simulink model "LAB2_1"  (R2025b)
settings: Solver=FixedStepAuto  StartTime=0.0  StopTime=5  FixedStep=0.0001  RelTol=1e-3
undefined symbols (not defined in the file): Beq, daq, DiscIntNeverNeededParam, drv, gbox, Jeq, Kd, Kp, mot, rads2rpm, Req, sens, T, tau_sf_est, Tl
settings Model: Creator=Gioele  LastModifiedBy=Gioele
settings DebuggingCC: MultiTaskCondExecSysMsg=warning  MultiTaskRateTransMsg=warning

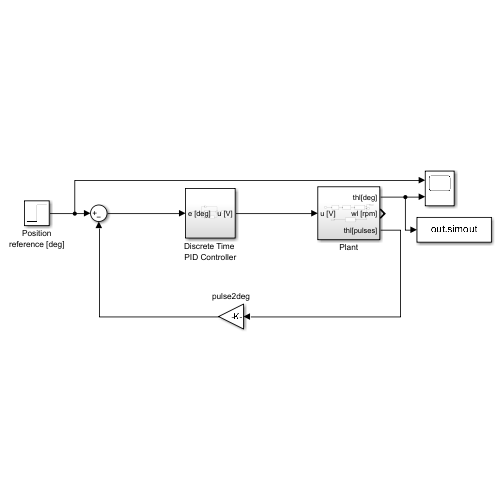
[thumbnail: Simulink's stored preview of the top-level diagram]
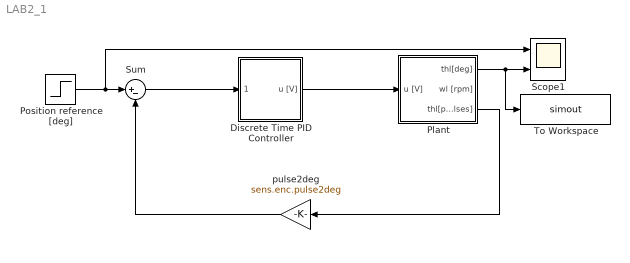
== system LAB2_1 ==
  Discrete Time PID Controller : Subsystem
  Plant : Subsystem
  Position reference [deg] : Step  Time=0  After=50  SampleTime=T
  Scope1 : Scope  NumInputPorts=2
      settings: ActiveDisplayYMinimum=40.583283463439479  ActiveDisplayYMaximum=71.669907924770413
  Sum : Sum  Inputs=|+-
  To Workspace : ToWorkspace  VariableName=simout  SampleTime=T
  pulse2deg : Gain  Gain=sens.enc.pulse2deg
  wires:
  Sum/1 -> Discrete Time PID Controller/1(e [deg])
  pulse2deg/1 -> Sum/2
  Plant/1(thl[deg]) -> To Workspace/1, Scope1/2
  Plant/3(thl[pulses]) -> pulse2deg/1
  Position reference [deg]/1 -> Scope1/1, Sum/1
  Discrete Time PID Controller/1(u [V]) -> Plant/1(u [V])

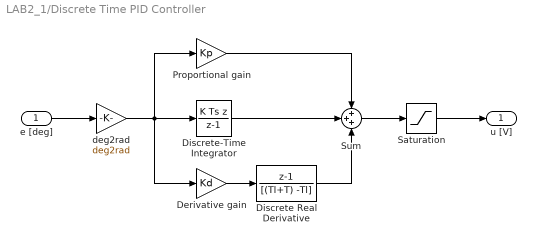
== system LAB2_1/Discrete Time PID Controller ==
  e [deg] : Inport
  Derivative gain : Gain  Gain=Kd
  Discrete Real Derivative : DiscreteTransferFcn  Numerator=[1 -1]  Denominator=[(Tl+T) -Tl]
  Discrete-Time Integrator : DiscreteIntegrator  IntegratorMethod=Integration: Backward Euler  gainval=Ki  SampleTime=T  ICPrevOutput=DiscIntNeverNeededParam  ICPrevScaledInput=DiscIntNeverNeededParam
  Proportional gain : Gain  Gain=Kp
  Saturation : Saturate  UpperLimit=daq.dac.fs  LowerLimit=-daq.dac.fs
  Sum : Sum  Inputs=+++
  deg2rad : Gain  Gain=deg2rad
  u [V] : Outport
  wires:
  Discrete Real Derivative/1 -> Sum/3
  Proportional gain/1 -> Sum/1
  e [deg]/1 -> deg2rad/1
  Sum/1 -> Saturation/1
  Saturation/1 -> u [V]/1
  deg2rad/1 -> Discrete-Time Integrator/1, Proportional gain/1, Derivative gain/1
  Derivative gain/1 -> Discrete Real Derivative/1
  Discrete-Time Integrator/1 -> Sum/2

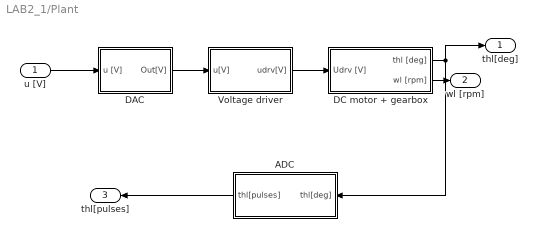
== system LAB2_1/Plant ==
  u [V] : Inport
  ADC : Subsystem  TreatAsAtomicUnit=on
  DAC : Subsystem  TreatAsAtomicUnit=on
  DC motor + gearbox : Subsystem
  Voltage driver : Subsystem  TreatAsAtomicUnit=on
  thl[deg] : Outport
  wl [rpm] : Outport  Port=2
  thl[pulses] : Outport  Port=3
  wires:
  Voltage driver/1(udrv[V]) -> DC motor + gearbox/1(Udrv [V])
  DC motor + gearbox/2(wl [rpm]) -> wl [rpm]/1
  DAC/1(Out[V]) -> Voltage driver/1(u[V])
  DC motor + gearbox/1(thl [deg]) -> thl[deg]/1, ADC/1(thl[deg])
  u [V]/1 -> DAC/1(u [V])
  ADC/1(thl[pulses]) -> thl[pulses]/1

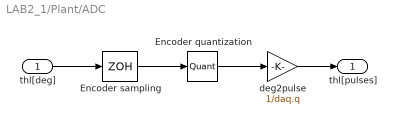
== system LAB2_1/Plant/ADC ==
  thl[deg] : Inport
  Encoder quantization : Quantizer  QuantizationInterval=daq.q
  Encoder sampling : ZeroOrderHold  SampleTime=0.001
  deg2pulse : Gain  Gain=1/daq.q
  thl[pulses] : Outport
  wires:
  Encoder quantization/1 -> deg2pulse/1
  thl[deg]/1 -> Encoder sampling/1
  Encoder sampling/1 -> Encoder quantization/1
  deg2pulse/1 -> thl[pulses]/1

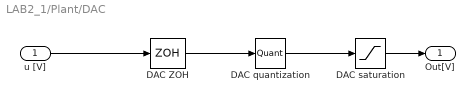
== system LAB2_1/Plant/DAC ==
  u [V] : Inport
  "DAC ZOH " : ZeroOrderHold  SampleTime=0.001
  DAC quantization : Quantizer  QuantizationInterval=daq.dac.q
  DAC saturation : Saturate  UpperLimit=daq.dac.fs  LowerLimit=-daq.dac.fs
  Out[V] : Outport
  wires:
  DAC quantization/1 -> DAC saturation/1
  u [V]/1 -> "DAC ZOH "/1
  "DAC ZOH "/1 -> DAC quantization/1
  DAC saturation/1 -> Out[V]/1

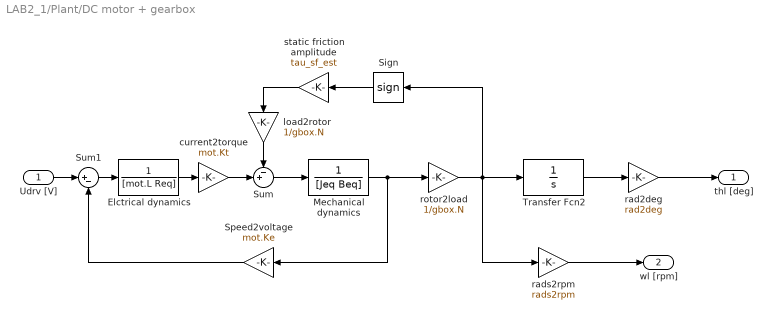
== system LAB2_1/Plant/DC motor + gearbox ==
  Udrv [V] : Inport
  Elctrical dynamics : TransferFcn  Denominator=[mot.L Req]
  Mechanical dynamics : TransferFcn  Denominator=[Jeq Beq]
  Sign : Signum  ZeroCross=off
  Speed2voltage : Gain  Gain=mot.Ke
  Sum : Sum  Inputs=-+|
  Sum1 : Sum  Inputs=|+-
  Transfer Fcn2 : TransferFcn  Denominator=[1 0]
  current2torque : Gain  Gain=mot.Kt
  load2rotor : Gain  Gain=1/gbox.N
  rad2deg : Gain  Gain=rad2deg
  rads2rpm : Gain  Gain=rads2rpm
  rotor2load : Gain  Gain=1/gbox.N
  static friction amplitude : Gain  Gain=tau_sf_est
  thl [deg] : Outport
  wl [rpm] : Outport  Port=2
  wires:
  rotor2load/1 -> Sign/1, rads2rpm/1, Transfer Fcn2/1
  Sign/1 -> static friction amplitude/1
  rads2rpm/1 -> wl [rpm]/1
  Sum/1 -> Mechanical dynamics/1
  Udrv [V]/1 -> Sum1/1
  static friction amplitude/1 -> load2rotor/1
  load2rotor/1 -> Sum/1
  Transfer Fcn2/1 -> rad2deg/1
  current2torque/1 -> Sum/2
  Speed2voltage/1 -> Sum1/2
  Mechanical dynamics/1 -> Speed2voltage/1, rotor2load/1
  Elctrical dynamics/1 -> current2torque/1
  Sum1/1 -> Elctrical dynamics/1
  rad2deg/1 -> thl [deg]/1

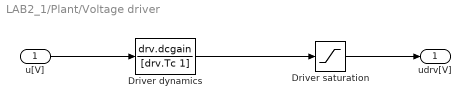
== system LAB2_1/Plant/Voltage driver ==
  u[V] : Inport
  Driver dynamics : TransferFcn  Numerator=drv.dcgain  Denominator=[drv.Tc 1]
  Driver saturation : Saturate  UpperLimit=drv.outmax  LowerLimit=-drv.outmax
  udrv[V] : Outport
  wires:
  Driver dynamics/1 -> Driver saturation/1
  u[V]/1 -> Driver dynamics/1
  Driver saturation/1 -> udrv[V]/1
